simulink model "forward_dynamics_test"  (R2024b)
settings: Solver=ode1  StartTime=0.0  StopTime=10.0  FixedStep=1e-3  RelTol=1e-3
libraries: sdu_controllers x2
settings Model: Creator=eld  LastModifiedBy=eld

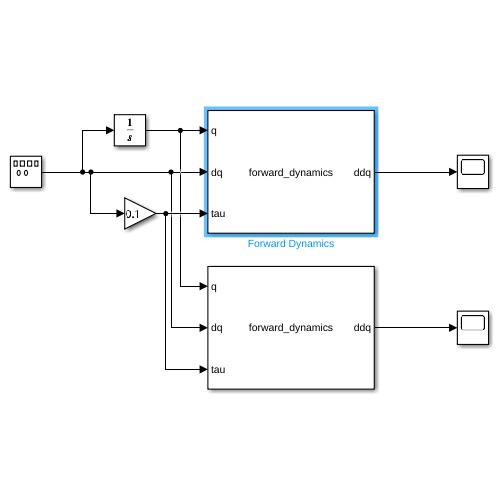
[thumbnail: Simulink's stored preview of the top-level diagram]
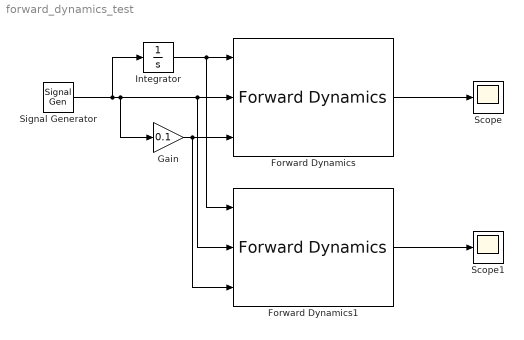
== system forward_dynamics_test ==
  Forward Dynamics : sdu_controllers/Forward Dynamics  RobotType=UR3e  SimulateUsing=Interpreted execution
  Forward Dynamics1 : sdu_controllers/Forward Dynamics  RobotType=UR5e  SimulateUsing=Interpreted execution
  Gain : Gain  Gain=0.1
  Integrator : Integrator
  Scope : Scope
  Scope1 : Scope
  Signal Generator : SignalGenerator  Amplitude=1 * ones(6,1)  Frequency=1 * ones(6,1)  Units=rad/sec
  wires:
  Signal Generator/1 -> Integrator/1, Gain/1, Forward Dynamics1/2, Forward Dynamics/2
  Integrator/1 -> Forward Dynamics1/1, Forward Dynamics/1
  Gain/1 -> Forward Dynamics1/3, Forward Dynamics/3
  Forward Dynamics/1 -> Scope/1
  Forward Dynamics1/1 -> Scope1/1
